simulink model "Lab9p1"  (R2024a)
settings: Solver=VariableStepAuto  StartTime=0.0  StopTime=100  RelTol=1e-3
libraries: simulink x1
settings Model: Creator=giuse  LastModifiedBy=giuse

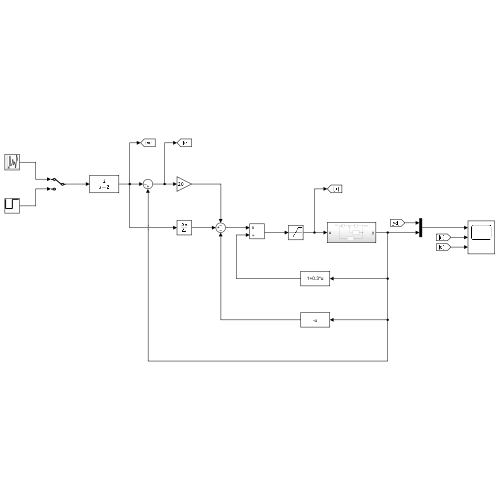
[thumbnail: Simulink's stored preview of the top-level diagram]
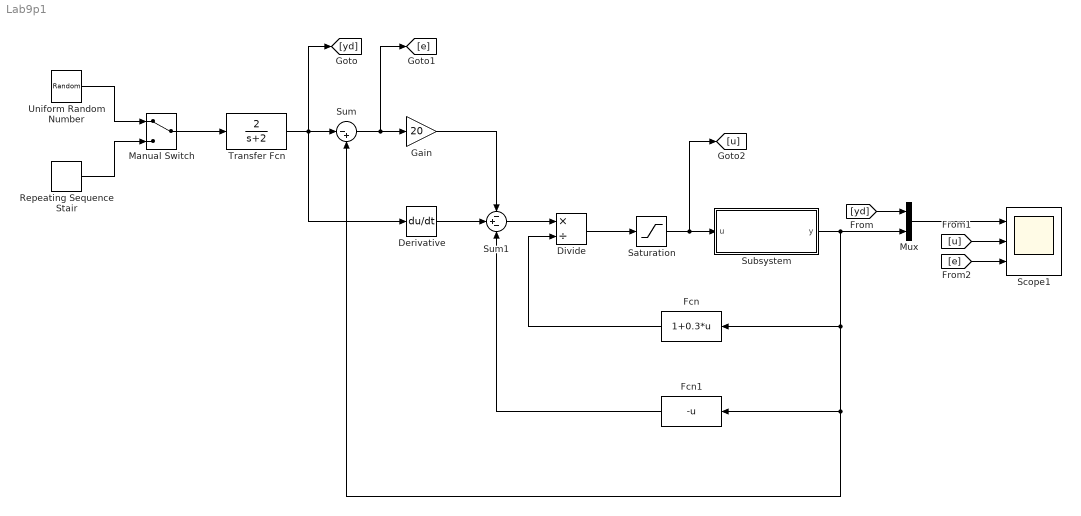
== system Lab9p1 ==
  Derivative : Derivative
  Divide : Product  Inputs=*/
  Fcn : Fcn  Expr=1+0.3*u
  Fcn1 : Fcn  Expr=-u
  Gain : Gain  Gain=20
  Manual Switch : ManualSwitch
  Mux : Mux  Inputs=2
  Repeating Sequence Stair : simulink/Sources/Repeating Sequence Stair  OutValues=[20 60].'  tsamp=10  OutMin=[]  OutMax=[]  OutDataTypeStr=double  OutputDataTypeScalingMode=double  OutDataType=fixdt(0,8)  ConRadixGroup=Best Precision: Vector-wise  OutScaling=2^-12
  Saturation : Saturate  UpperLimit=10  LowerLimit=-10
  Scope1 : Scope  NumInputPorts=3
  Subsystem : Subsystem
  Sum : Sum  Inputs=|-+
  Sum1 : Sum  Inputs=-+-
  Transfer Fcn : TransferFcn  Numerator=[2]  Denominator=[1 2]
  Uniform Random Number : UniformRandomNumber  Minimum=20  Maximum=60  SampleTime=10
  wires:
  Uniform Random Number/1 -> Manual Switch/1
  Repeating Sequence Stair/1 -> Manual Switch/2
  Manual Switch/1 -> Transfer Fcn/1
  Transfer Fcn/1 -> [yd], Derivative/1, Sum/1
  Sum/1 -> [e], Gain/1
  Gain/1 -> Sum1/1
  Derivative/1 -> Sum1/2
  Sum1/1 -> Divide/1
  Divide/1 -> Saturation/1
  Saturation/1 -> [u], Subsystem/1(u)
  Fcn/1 -> Divide/2
  Fcn1/1 -> Sum1/3
  Subsystem/1(y) -> Sum/2, Fcn1/1, Fcn/1, Mux/2
  Mux/1 -> Scope1/1
  [yd] -> Mux/1
  [u] -> Scope1/2
  [e] -> Scope1/3

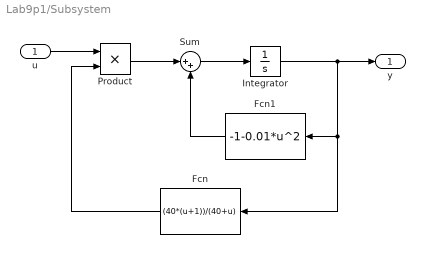
== system Lab9p1/Subsystem ==
  u : Inport
  Fcn : Fcn  Expr=(40*(u+1))/(40+u)
  Fcn1 : Fcn  Expr=-1-0.01*u^2
  Integrator : Integrator
  Product : Product
  Sum : Sum  Inputs=|++
  y : Outport
  wires:
  u/1 -> Product/1
  Fcn/1 -> Product/2
  Product/1 -> Sum/1
  Fcn1/1 -> Sum/2
  Sum/1 -> Integrator/1
  Integrator/1 -> Fcn/1, Fcn1/1, y/1
